simulink model "call_ode_spmet_cccv"  (R2019a)
settings: Solver=VariableStepAuto  StartTime=0.0  StopTime=10.0  RelTol=1e-3
undefined symbols (not defined in the file or in its folder): x0_nom
settings Model: Creator=ztakeo  LastModifiedBy=ztakeo

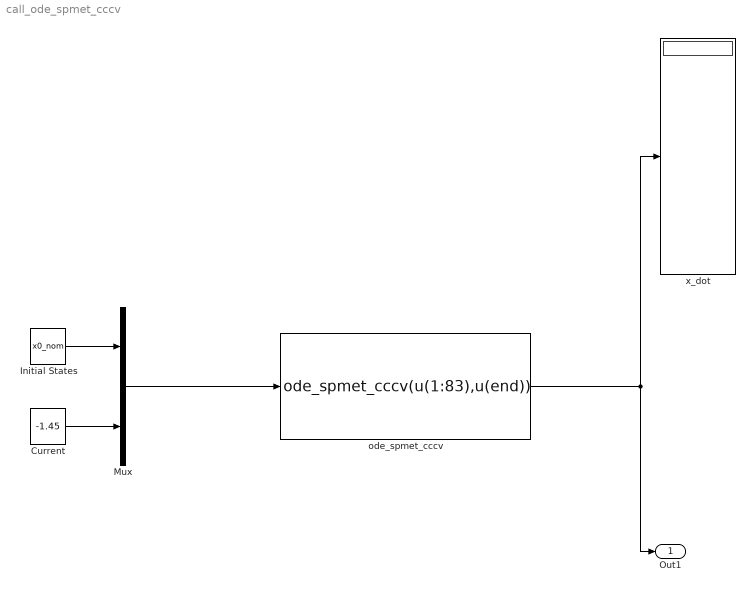
== system call_ode_spmet_cccv ==
  "Current " : Constant  Value=-1.45
  Initial States : Constant  Value=x0_nom
  Mux : Mux  Inputs=2
  ode_spmet_cccv : MATLABFcn  MATLABFcn=ode_spmet_cccv(u(1:83),u(end))
  x_dot : Display
  Out1 : Outport
  wires:
  Mux/1 -> ode_spmet_cccv/1
  Initial States/1 -> Mux/1
  "Current "/1 -> Mux/2
  ode_spmet_cccv/1 -> Out1/1, x_dot/1
